simulink model "simulator_manual_MPC"  (R2025b)
settings: Solver=FixedStepAuto  StartTime=0.0  StopTime=100  FixedStep=0.01  RelTol=1e-3
values from neighbouring files (symbols this model uses):
  q0 = [0; 0; 0]    [model_init.m]    (also in test_model.m = x_test(1:3))
  qdot0 = [0;0;0]    [model_init.m]
  W_inv = inv(system_params.W)    [model_init.m]
undefined symbols (not defined in the file or in its folder): MPC_settings, P0, Q_kf, R_kf, system_params, x0
libraries: slpidlib x5
settings Model: Creator=Sigbjørn  LastModifiedBy=sig

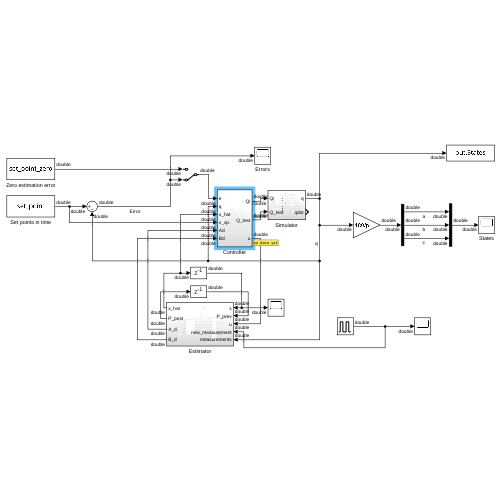
[thumbnail: Simulink's stored preview of the top-level diagram]
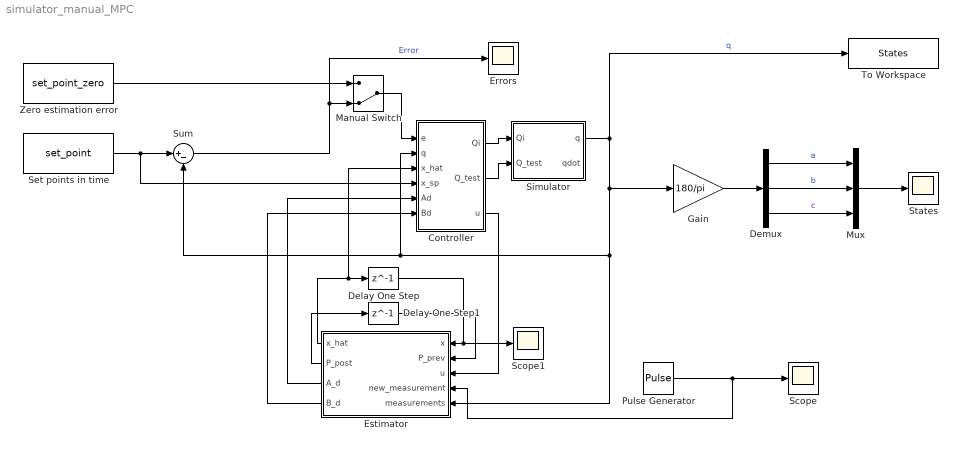
== system simulator_manual_MPC ==
  Controller : Subsystem
  Delay One Step : Delay  DelayLength=1  InitialCondition=x0
  Delay One Step1 : Delay  DelayLength=1  InitialCondition=P0
  Demux : Demux  Outputs=3
  Errors : Scope
      settings: ActiveDisplayYMinimum=-1.818734816898053E+64  ActiveDisplayYMaximum=2.7677532819561327E+63
  Estimator : Subsystem
      settings: PortSchema="{\"entries\":[{\"content\":{\"sides\":[{\"content\":{\"connectorIds\":[\"Out1\",\"Out2\",\"Out3\",\"Out4\"]},\"type\":\"ConnectorPlacement.EquallySpacedRectSide\",\"uuid\":\"f477ef40-4352-4d84-a45f-d7b8149414e1\"},{\"content\":{\"connectorIds\":[\"In1\",\"In2\",\"In3\",\"In4\",\"In5\"],\"side\":\"RIGHT\"},\"type\":\"ConnectorPlacement.EquallySpacedRectSide\",\"uuid\":\"8f29c47b-7819-47b7-a7db-3d460012710f\"},{\"content\":{\"side\":\"TOP\"},\"type\":\"ConnectorPlacement.EquallySpacedRectSide\",\"uuid\":\"6fcef62b-5cfa-49ba-93f4-5d540223ca0d\"}]},\"type\":\"ConnectorPlacement.EquallySpacedConnector\",\"uuid\":\"aa31ebfc-db05-4e23-be25-e9e271d34221\"}],\"packageUris\":[\"http://schema.mathworks.com/mf0/Connector/R2020b\"],\"version\":\"1.0\"}"
  Gain : Gain  Gain=180/pi
  Manual Switch : ManualSwitch  CurrentSetting=0
  Mux : Mux  Inputs=3
  Pulse Generator : DiscretePulseGenerator  PulseType=Time based  Period=0.1  PulseWidth=10
  Scope : Scope
      settings: ActiveDisplayYMinimum=-0.12499999999999997  ActiveDisplayYMaximum=1.125  DataLoggingVariableName=ScopeData11
  Scope1 : Scope
      settings: ActiveDisplayYMinimum=-0.00092258079795706066  ActiveDisplayYMaximum=0.0024721822800288758  DataLoggingVariableName=ScopeData13
  Set points in time : FromWorkspace  VariableName=set_point
  Simulator : Subsystem
  States : Scope
      settings: ActiveDisplayYMinimum=-1.5858058178956856E+65  ActiveDisplayYMaximum=1.0420582906175698E+66
  Sum : Sum  Inputs=|+-
  To Workspace : ToWorkspace  VariableName=States  SaveFormat=Timeseries  SampleTime=-1
  Zero estimation error : FromWorkspace  VariableName=set_point_zero
  wires:
  Controller/1(Qi) -> Simulator/1(Qi)
  Sum/1 -> Manual Switch/2, Errors/1  "Error"
  Simulator/1(q) -> Estimator/5(measurements), Controller/2(q), Sum/2, Gain/1, To Workspace/1  "q"
  Demux/1 -> Mux/1  "a"
  Demux/2 -> Mux/2  "b"
  Demux/3 -> Mux/3  "c"
  Zero estimation error/1 -> Manual Switch/1
  Manual Switch/1 -> Controller/1(e)
  Gain/1 -> Demux/1
  Mux/1 -> States/1
  Controller/2(Q_test) -> Simulator/2(Q_test)
  Controller/3(u) -> Estimator/3(u)
  Pulse Generator/1 -> Estimator/4(new_measurement), Scope/1
  Estimator/1(x_hat) -> Controller/3(x_hat), Delay One Step/1
  Estimator/2(P_post) -> Delay One Step1/1
  Delay One Step/1 -> Scope1/1, Estimator/1(x)
  Delay One Step1/1 -> Estimator/2(P_prev)
  Estimator/3(A_d) -> Controller/5(Ad)
  Estimator/4(B_d) -> Controller/6(Bd)
  Set points in time/1 -> Controller/4(x_sp), Sum/1

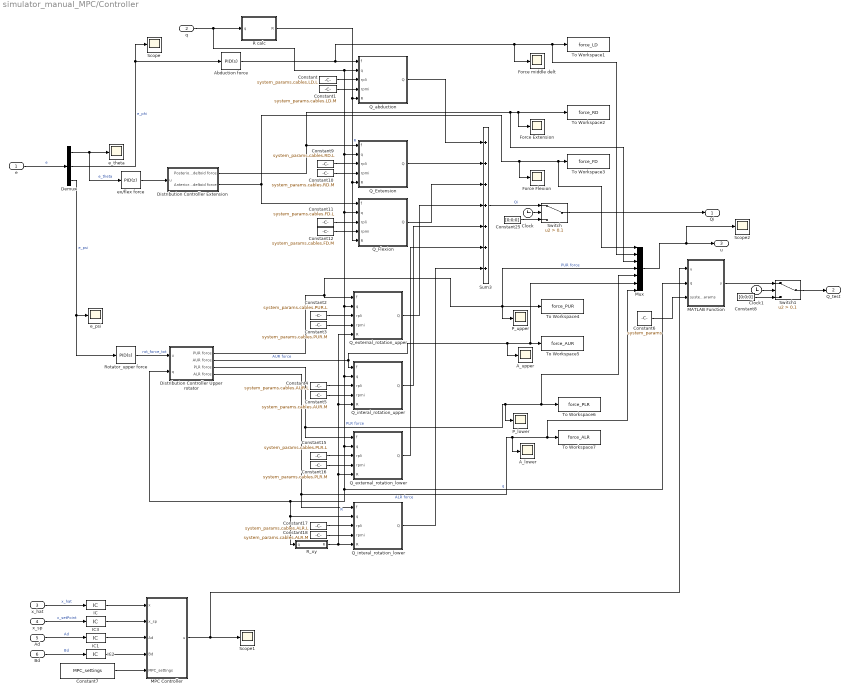
== system simulator_manual_MPC/Controller ==
  e : Inport
  q : Inport  Port=2
  x_hat : Inport  Port=3
  x_sp : Inport  Port=4
  Ad : Inport  Port=5
  Bd : Inport  Port=6
  A_lower : Scope
      settings: ActiveDisplayYMinimum=-66.70773  ActiveDisplayYMaximum=600.36959  DataLoggingVariableName=ScopeData3
  A_upper : Scope
      settings: ActiveDisplayYMinimum=-10.373094653487385  ActiveDisplayYMaximum=93.35785188138648  DataLoggingVariableName=ScopeData4
  Abduction force : slpidlib/PID Controller  Controller=PID  Form=Parallel  TimeDomain=Continuous-time  UseExternalTs=off  SampleTime=-1  IntegratorMethod=Forward Euler  FilterMethod=Forward Euler  ControllerParametersSource=internal  P=1  I=25  UseKiTs=off  D=5  UseExternalDerivativeSource=off  N=100  UseFilter=on  TunerSelectOption=Transfer Function Based (PID Tuner App)  InitialConditionSource=internal  InitialConditionForIntegrator=0  InitialConditionForFilter=0  DifferentiatorICPrevScaledInput=0  ExternalReset=none  TrackingMode=off  Kt=1  LimitOutput=on  SatLimitsSource=internal  UpperSaturationLimit=inf  LowerSaturationLimit=0  LinearizeAsGain=on  AntiWindupMode=none  Kb=1  LimitIntegrator=on  UpperIntegratorSaturationLimit=10000  LowerIntegratorSaturationLimit=0  POutMin=[]  POutMax=[]  IOutMin=[]  IOutMax=[]  DOutMin=[]  DOutMax=[]  NOutMin=[]  NOutMax=[]  SumOutMin=[]  SumOutMax=[]  SaturationOutMin=[]  SaturationOutMax=[]  PParamMin=[]  PParamMax=[]  IParamMin=[]  IParamMax=[]  DParamMin=[]  DParamMax=[]  NParamMin=[]  NParamMax=[]  KbParamMin=[]  KbParamMax=[]  KtParamMin=[]  KtParamMax=[]  KbOutMin=[]  KbOutMax=[]  KtOutMin=[]  KtOutMax=[]  IntegratorOutMin=[]  IntegratorOutMax=[]  FilterOutMin=[]  FilterOutMax=[]  SumI1OutMin=[]  SumI1OutMax=[]  SumI2OutMin=[]  SumI2OutMax=[]  SumI3OutMin=[]  SumI3OutMax=[]  SumI4OutMin=[]  SumI4OutMax=[]  SumDOutMin=[]  SumDOutMax=[]  DifferentiatorOutMin=[]  DifferentiatorOutMax=[]  FilterDiffOutCoefMin=[]  FilterDiffOutCoefMax=[]  ReciprocalOutMin=[]  ReciprocalOutMax=[]  SumDenOutMin=[]  SumDenOutMax=[]  SumNumOutMin=[]  SumNumOutMax=[]  DivideOutMin=[]  DivideOutMax=[]  UdiffTsProdOutMin=[]  UdiffTsProdOutMax=[]  NTsProdOutMin=[]  NTsProdOutMax=[]  UintegralTsProdOutMin=[]  UintegralTsProdOutMax=[]  UngainTsProdOutMin=[]  UngainTsProdOutMax=[]  ClampingZeroOutDataTypeStr=Inherit: Inherit via back propagation  ClampingZeroOutMin=[]  ClampingZeroOutMax=[]  FilterDenConstantOutDataTypeStr=Inherit: Inherit via back propagation  FilterDenConstantOutMin=[]  FilterDenConstantOutMax=[]  PCopyOutDataTypeStr=Inherit: Inherit via back propagation  PCopyOutMin=[]  PCopyOutMax=[]  NCopyOutDataTypeStr=Inherit: Inherit via back propagation  NCopyOutMin=[]  NCopyOutMax=[]  IntegratorContinuousStateAttributes=''  IntegratorStateMustResolveToSignalObject=off  IntegratorRTWStateStorageClass=Auto  FilterContinuousStateAttributes=''  FilterStateMustResolveToSignalObject=off  FilterRTWStateStorageClass=Auto  ParallelPVariant=InternalParameters  IdealPVariant=Disabled  IVariant=InternalParameters  DVariant=InternalParameters  IntegratorVariant=Continuous  SatVariant=Enabled  AWVariant=Passthrough  PCopyVariant=Disabled  TRVariant=Disabled  FdbkBlocksVariant=Forward  IdealPFdbkVariant=Disabled  SatFdbkVariant=Disabled  DerivativeFilterVariant=ContFilter  NVariant=InternalParameters  NCopyVariant=Disabled  FilterICVariant=InternalICsFilter  IntegratorICVariant=InternalICs  ExternalResetVariant=Disabled  TRSumVariant=Passthrough  SumFdbkVariant=Disabled  SumVariant=Sum_PID  TsampFilterVariant=InternalTs  TsampNgainVariant=Passthrough  TsampIntegralVariant=Disabled_SignalSpec  ExternalSaturationOutDataTypeStr=Inherit: Same as second input  DerivativeSourceVariant=ErrorSignal  PreIntVariant=InternalPreInt
  Clock : Clock
  Clock1 : Clock
  Constant : Constant  Value=system_params.cables.LD.L
  Constant1 : Constant  Value=system_params.cables.LD.M
  Constant10 : Constant  Value=system_params.cables.RD.M
  Constant11 : Constant  Value=system_params.cables.FD.L
  Constant12 : Constant  Value=system_params.cables.FD.M
  Constant15 : Constant  Value=system_params.cables.PLR.L
  Constant16 : Constant  Value=system_params.cables.PLR.M
  Constant17 : Constant  Value=system_params.cables.ALR.L
  Constant18 : Constant  Value=system_params.cables.ALR.M
  Constant2 : Constant  Value=system_params.cables.PUR.L
  Constant25 : Constant  Value=[0;0;0]
  Constant3 : Constant  Value=system_params.cables.PUR.M
  Constant4 : Constant  Value=system_params.cables.AUR.L
  Constant5 : Constant  Value=system_params.cables.AUR.M
  Constant6 : Constant  Value=system_params  OutDataTypeStr=Bus: System_params_bus
  Constant7 : Constant  Value=MPC_settings  OutDataTypeStr=Bus: MPCBus
  Constant8 : Constant  Value=[0;0;0]
  Constant9 : Constant  Value=system_params.cables.RD.L
  Demux : Demux  Outputs=3
  Distribution Controller Extension : Subsystem
  Distribution Controller Upper rotator : Subsystem
  Force Extension : Scope
      settings: ActiveDisplayYMinimum=-60.902718832950853  ActiveDisplayYMaximum=560.55994041701729
  Force Flexion : Scope
      settings: ActiveDisplayYMinimum=-3.2054062543658342  ActiveDisplayYMaximum=29.503154758790387  DataLoggingVariableName=ScopeData2
  Force middle delt : Scope
      settings: ActiveDisplayYMinimum=-835.43898  ActiveDisplayYMaximum=7657.08353  DataLoggingVariableName=ScopeData3
  IC : InitialCondition  Value=x0
  IC1 : InitialCondition  Value=zeros(6,6)
  IC2 : InitialCondition  Value=zeros(6,7)
  IC3 : InitialCondition  Value=zeros(3,1)
  MATLAB Function : MATLAB Function  TreatAsAtomicUnit=on
  MPC Controller : MATLAB Function  TreatAsAtomicUnit=on
  Mux : Mux  Inputs=7
  P_lower : Scope
      settings: ActiveDisplayYMinimum=-3.51093  ActiveDisplayYMaximum=31.5984  DataLoggingVariableName=ScopeData2
  P_upper : Scope
      settings: ActiveDisplayYMinimum=-0.42649  ActiveDisplayYMaximum=3.83839
  Q_Extension : MATLAB Function  TreatAsAtomicUnit=on
  Q_Flexion : MATLAB Function  TreatAsAtomicUnit=on
  Q_abduction : MATLAB Function  TreatAsAtomicUnit=on
  Q_external_rotation_lower : MATLAB Function  TreatAsAtomicUnit=on
  Q_external_rotation_upper : MATLAB Function  TreatAsAtomicUnit=on
  Q_interal_rotation_lower : MATLAB Function  TreatAsAtomicUnit=on
  Q_interal_rotation_upper : MATLAB Function  TreatAsAtomicUnit=on
  R calc : MATLAB Function  TreatAsAtomicUnit=on
  R_xy : MATLAB Function  TreatAsAtomicUnit=on
  Rotator_upper force : slpidlib/PID Controller  Controller=PID  Form=Parallel  TimeDomain=Continuous-time  UseExternalTs=off  SampleTime=-1  IntegratorMethod=Forward Euler  FilterMethod=Forward Euler  ControllerParametersSource=internal  P=100  I=200  UseKiTs=off  D=500  UseExternalDerivativeSource=off  N=100  UseFilter=on  TunerSelectOption=Transfer Function Based (PID Tuner App)  InitialConditionSource=internal  InitialConditionForIntegrator=0  InitialConditionForFilter=0  DifferentiatorICPrevScaledInput=0  ExternalReset=none  TrackingMode=off  Kt=1  LimitOutput=on  SatLimitsSource=internal  UpperSaturationLimit=inf  LowerSaturationLimit=-inf  LinearizeAsGain=on  AntiWindupMode=none  Kb=1  LimitIntegrator=on  UpperIntegratorSaturationLimit=inf  LowerIntegratorSaturationLimit=-inf  POutMin=[]  POutMax=[]  IOutMin=[]  IOutMax=[]  DOutMin=[]  DOutMax=[]  NOutMin=[]  NOutMax=[]  SumOutMin=[]  SumOutMax=[]  SaturationOutMin=[]  SaturationOutMax=[]  PParamMin=[]  PParamMax=[]  IParamMin=[]  IParamMax=[]  DParamMin=[]  DParamMax=[]  NParamMin=[]  NParamMax=[]  KbParamMin=[]  KbParamMax=[]  KtParamMin=[]  KtParamMax=[]  KbOutMin=[]  KbOutMax=[]  KtOutMin=[]  KtOutMax=[]  IntegratorOutMin=[]  IntegratorOutMax=[]  FilterOutMin=[]  FilterOutMax=[]  SumI1OutMin=[]  SumI1OutMax=[]  SumI2OutMin=[]  SumI2OutMax=[]  SumI3OutMin=[]  SumI3OutMax=[]  SumI4OutMin=[]  SumI4OutMax=[]  SumDOutMin=[]  SumDOutMax=[]  DifferentiatorOutMin=[]  DifferentiatorOutMax=[]  FilterDiffOutCoefMin=[]  FilterDiffOutCoefMax=[]  ReciprocalOutMin=[]  ReciprocalOutMax=[]  SumDenOutMin=[]  SumDenOutMax=[]  SumNumOutMin=[]  SumNumOutMax=[]  DivideOutMin=[]  DivideOutMax=[]  UdiffTsProdOutMin=[]  UdiffTsProdOutMax=[]  NTsProdOutMin=[]  NTsProdOutMax=[]  UintegralTsProdOutMin=[]  UintegralTsProdOutMax=[]  UngainTsProdOutMin=[]  UngainTsProdOutMax=[]  ClampingZeroOutDataTypeStr=Inherit: Inherit via back propagation  ClampingZeroOutMin=[]  ClampingZeroOutMax=[]  FilterDenConstantOutDataTypeStr=Inherit: Inherit via back propagation  FilterDenConstantOutMin=[]  FilterDenConstantOutMax=[]  PCopyOutDataTypeStr=Inherit: Inherit via back propagation  PCopyOutMin=[]  PCopyOutMax=[]  NCopyOutDataTypeStr=Inherit: Inherit via back propagation  NCopyOutMin=[]  NCopyOutMax=[]  IntegratorContinuousStateAttributes=''  IntegratorStateMustResolveToSignalObject=off  IntegratorRTWStateStorageClass=Auto  FilterContinuousStateAttributes=''  FilterStateMustResolveToSignalObject=off  FilterRTWStateStorageClass=Auto  ParallelPVariant=InternalParameters  IdealPVariant=Disabled  IVariant=InternalParameters  DVariant=InternalParameters  IntegratorVariant=Continuous  SatVariant=Enabled  AWVariant=Passthrough  PCopyVariant=Disabled  TRVariant=Disabled  FdbkBlocksVariant=Forward  IdealPFdbkVariant=Disabled  SatFdbkVariant=Disabled  DerivativeFilterVariant=ContFilter  NVariant=InternalParameters  NCopyVariant=Disabled  FilterICVariant=InternalICsFilter  IntegratorICVariant=InternalICs  ExternalResetVariant=Disabled  TRSumVariant=Passthrough  SumFdbkVariant=Disabled  SumVariant=Sum_PID  TsampFilterVariant=InternalTs  TsampNgainVariant=Passthrough  TsampIntegralVariant=Disabled_SignalSpec  ExternalSaturationOutDataTypeStr=Inherit: Same as second input  DerivativeSourceVariant=ErrorSignal  PreIntVariant=InternalPreInt
  Scope : Scope
      settings: ActiveDisplayYMinimum=-0.00043  ActiveDisplayYMaximum=5E-5  DataLoggingVariableName=ScopeData5
  Scope1 : Scope
      settings: ActiveDisplayYMinimum=-126637.74464504365  ActiveDisplayYMaximum=129137.74464504365  DataLoggingVariableName=ScopeData14
  Scope2 : Scope
      settings: ActiveDisplayYMinimum=-76.031922907283175  ActiveDisplayYMaximum=684.28730616554867  DataLoggingVariableName=ScopeData15
  Sum3 : Sum  Inputs=+++++++  InputSameDT=on  SaturateOnIntegerOverflow=on  OutDataTypeStr=Inherit: Same as first input
  Switch : Switch  Criteria=u2 > Threshold  Threshold=0.1  SaturateOnIntegerOverflow=off  InputSameDT=off
  Switch1 : Switch  Criteria=u2 > Threshold  Threshold=0.1  SaturateOnIntegerOverflow=off  InputSameDT=off
  To Workspace1 : ToWorkspace  VariableName=force_LD  SaveFormat=Timeseries  SampleTime=-1
  To Workspace2 : ToWorkspace  VariableName=force_RD  SaveFormat=Timeseries  SampleTime=-1
  To Workspace3 : ToWorkspace  VariableName=force_FD  SaveFormat=Timeseries  SampleTime=-1
  To Workspace4 : ToWorkspace  VariableName=force_PUR  SaveFormat=Timeseries  SampleTime=-1
  To Workspace5 : ToWorkspace  VariableName=force_AUR  SaveFormat=Timeseries  SampleTime=-1
  To Workspace6 : ToWorkspace  VariableName=force_PLR  SaveFormat=Timeseries  SampleTime=-1
  To Workspace7 : ToWorkspace  VariableName=force_ALR  SaveFormat=Timeseries  SampleTime=-1
  e_psi : Scope
      settings: ActiveDisplayYMinimum=-10.03144  ActiveDisplayYMaximum=67.48296  DataLoggingVariableName=ScopeData3
  e_theta : Scope
      settings: ActiveDisplayYMinimum=-0.00064  ActiveDisplayYMaximum=0.00057  DataLoggingVariableName=ScopeData6
  ex/flex force : slpidlib/PID Controller  Controller=PID  Form=Parallel  TimeDomain=Discrete-time  UseExternalTs=off  SampleTime=-1  IntegratorMethod=Forward Euler  FilterMethod=Forward Euler  ControllerParametersSource=internal  P=1  I=25  UseKiTs=off  D=5  UseExternalDerivativeSource=off  N=100  UseFilter=on  TunerSelectOption=Transfer Function Based (PID Tuner App)  InitialConditionSource=internal  InitialConditionForIntegrator=0  InitialConditionForFilter=0  DifferentiatorICPrevScaledInput=0  ExternalReset=none  TrackingMode=off  Kt=1  LimitOutput=on  SatLimitsSource=internal  UpperSaturationLimit=inf  LowerSaturationLimit=-inf  LinearizeAsGain=on  AntiWindupMode=none  Kb=1  LimitIntegrator=on  UpperIntegratorSaturationLimit=inf  LowerIntegratorSaturationLimit=-inf  POutMin=[]  POutMax=[]  IOutMin=[]  IOutMax=[]  DOutMin=[]  DOutMax=[]  NOutMin=[]  NOutMax=[]  SumOutMin=[]  SumOutMax=[]  SaturationOutMin=[]  SaturationOutMax=[]  PParamMin=[]  PParamMax=[]  IParamMin=[]  IParamMax=[]  DParamMin=[]  DParamMax=[]  NParamMin=[]  NParamMax=[]  KbParamMin=[]  KbParamMax=[]  KtParamMin=[]  KtParamMax=[]  KbOutMin=[]  KbOutMax=[]  KtOutMin=[]  KtOutMax=[]  IntegratorOutMin=[]  IntegratorOutMax=[]  FilterOutMin=[]  FilterOutMax=[]  SumI1OutMin=[]  SumI1OutMax=[]  SumI2OutMin=[]  SumI2OutMax=[]  SumI3OutMin=[]  SumI3OutMax=[]  SumI4OutMin=[]  SumI4OutMax=[]  SumDOutMin=[]  SumDOutMax=[]  DifferentiatorOutMin=[]  DifferentiatorOutMax=[]  FilterDiffOutCoefMin=[]  FilterDiffOutCoefMax=[]  ReciprocalOutMin=[]  ReciprocalOutMax=[]  SumDenOutMin=[]  SumDenOutMax=[]  SumNumOutMin=[]  SumNumOutMax=[]  DivideOutMin=[]  DivideOutMax=[]  UdiffTsProdOutMin=[]  UdiffTsProdOutMax=[]  NTsProdOutMin=[]  NTsProdOutMax=[]  UintegralTsProdOutMin=[]  UintegralTsProdOutMax=[]  UngainTsProdOutMin=[]  UngainTsProdOutMax=[]  ClampingZeroOutDataTypeStr=Inherit: Inherit via back propagation  ClampingZeroOutMin=[]  ClampingZeroOutMax=[]  FilterDenConstantOutDataTypeStr=Inherit: Inherit via back propagation  FilterDenConstantOutMin=[]  FilterDenConstantOutMax=[]  PCopyOutDataTypeStr=Inherit: Inherit via back propagation  PCopyOutMin=[]  PCopyOutMax=[]  NCopyOutDataTypeStr=Inherit: Inherit via back propagation  NCopyOutMin=[]  NCopyOutMax=[]  IntegratorContinuousStateAttributes=''  IntegratorStateMustResolveToSignalObject=off  IntegratorRTWStateStorageClass=Auto  FilterContinuousStateAttributes=''  FilterStateMustResolveToSignalObject=off  FilterRTWStateStorageClass=Auto  ParallelPVariant=InternalParameters  IdealPVariant=Disabled  IVariant=InternalParameters  DVariant=InternalParameters  IntegratorVariant=Discrete  SatVariant=Enabled  AWVariant=Passthrough  PCopyVariant=Disabled  TRVariant=Disabled  FdbkBlocksVariant=Forward  IdealPFdbkVariant=Disabled  SatFdbkVariant=Disabled  DerivativeFilterVariant=ForwardEulerFilter  NVariant=InternalParameters  NCopyVariant=Disabled  FilterICVariant=InternalICsFilter  IntegratorICVariant=InternalICs  ExternalResetVariant=Disabled  TRSumVariant=Passthrough  SumFdbkVariant=Disabled  SumVariant=Sum_PID  TsampFilterVariant=InternalTs  TsampNgainVariant=Passthrough  TsampIntegralVariant=Disabled_SignalSpec  ExternalSaturationOutDataTypeStr=Inherit: Same as second input  DerivativeSourceVariant=ErrorSignal  PreIntVariant=InternalPreInt
  Qi : Outport
  Q_test : Outport  Port=2
  u : Outport  Port=3
  wires:
  q/1 -> Q_abduction/2(q), Q_Extension/2(q), Q_Flexion/2(q), MATLAB Function/2(q), Q_interal_rotation_lower/2(q), R_xy/1(q), Distribution Controller Upper rotator/2(q), Q_external_rotation_lower/2(q), Q_interal_rotation_upper/2(q), Q_external_rotation_upper/2(q), R calc/1(q)  "q"
  R calc/1(R) -> Q_Extension/5(R), Q_Flexion/5(R), Q_abduction/5(R)  "R"
  Constant/1 -> Q_abduction/3(rpli)
  Constant1/1 -> Q_abduction/4(rpmi)
  Sum3/1 -> Switch/1  "Qi"
  Demux/1 -> ex/flex force/1, e_theta/1  "e_theta"
  Demux/2 -> Scope/1, Abduction force/1  "e_phi"
  Demux/3 -> Rotator_upper force/1, e_psi/1  "e_psi"
  Constant2/1 -> Q_external_rotation_upper/3(rpli)
  Constant3/1 -> Q_external_rotation_upper/4(rpmi)
  Constant4/1 -> Q_interal_rotation_upper/3(rpli)
  Constant5/1 -> Q_interal_rotation_upper/4(rpmi)
  Q_abduction/1(Q) -> Sum3/1
  Q_interal_rotation_upper/1(Q) -> Sum3/5
  Q_external_rotation_upper/1(Q) -> Sum3/4
  Rotator_upper force/1 -> Distribution Controller Upper rotator/1(u)  "rot_force_tot"
  ex/flex force/1 -> Distribution Controller Extension/1(u)
  Constant9/1 -> Q_Extension/3(rpli)
  Constant10/1 -> Q_Extension/4(rpmi)
  Constant11/1 -> Q_Flexion/3(rpli)
  Constant12/1 -> Q_Flexion/4(rpmi)
  Q_Flexion/1(Q) -> Sum3/3
  Q_Extension/1(Q) -> Sum3/2
  Abduction force/1 -> Force middle delt/1, Mux/2, To Workspace1/1, Q_abduction/1(f)
  Distribution Controller Extension/1(Posterior deltoid force) -> Mux/3, To Workspace2/1, Force Extension/1, Q_Extension/1(f)
  Distribution Controller Extension/2(Anterior deltoid force) -> Q_Flexion/1(f), Mux/1, To Workspace3/1, Force Flexion/1
  Q_external_rotation_lower/1(Q) -> Sum3/6
  Q_interal_rotation_lower/1(Q) -> Sum3/7
  Constant15/1 -> Q_external_rotation_lower/3(rpli)
  Constant16/1 -> Q_external_rotation_lower/4(rpmi)
  Constant17/1 -> Q_interal_rotation_lower/3(rpli)
  Constant18/1 -> Q_interal_rotation_lower/4(rpmi)
  e/1 -> Demux/1  "e"
  Clock/1 -> Switch/2
  Constant25/1 -> Switch/3
  Switch/1 -> Qi/1
  Distribution Controller Upper rotator/4(ALR force) -> Mux/7, To Workspace7/1, A_lower/1, Q_interal_rotation_lower/1(f)  "ALR force"
  Distribution Controller Upper rotator/3(PLR force) -> Mux/5, To Workspace6/1, P_lower/1, Q_external_rotation_lower/1(f)  "PLR force"
  Distribution Controller Upper rotator/2(AUR force) -> A_upper/1, Mux/6, To Workspace5/1, Q_interal_rotation_upper/1(f)  "AUR force"
  Distribution Controller Upper rotator/1(PUR force) -> Mux/4, To Workspace4/1, P_upper/1, Q_external_rotation_upper/1(f)  "PUR force"
  R_xy/1(R) -> Q_external_rotation_upper/5(R), Q_interal_rotation_upper/5(R), Q_external_rotation_lower/5(R), Q_interal_rotation_lower/5(R)  "R"
  Mux/1 -> Scope2/1, u/1
  MATLAB Function/1(y) -> Switch1/1
  Constant6/1 -> MATLAB Function/3(system_params)
  x_hat/1 -> IC/1  "x_hat"
  Ad/1 -> IC1/1  "Ad"
  Bd/1 -> IC2/1  "Bd"
  Constant7/1 -> MPC Controller/5(MPC_settings)
  MPC Controller/1(u) -> MATLAB Function/1(u), Scope1/1
  x_sp/1 -> IC3/1  "x_setPoint"
  Constant8/1 -> Switch1/3
  Switch1/1 -> Q_test/1
  Clock1/1 -> Switch1/2
  IC/1 -> MPC Controller/1(x)
  IC1/1 -> MPC Controller/3(Ad)
  IC2/1 -> MPC Controller/4(Bd)
  IC3/1 -> MPC Controller/2(x_sp)

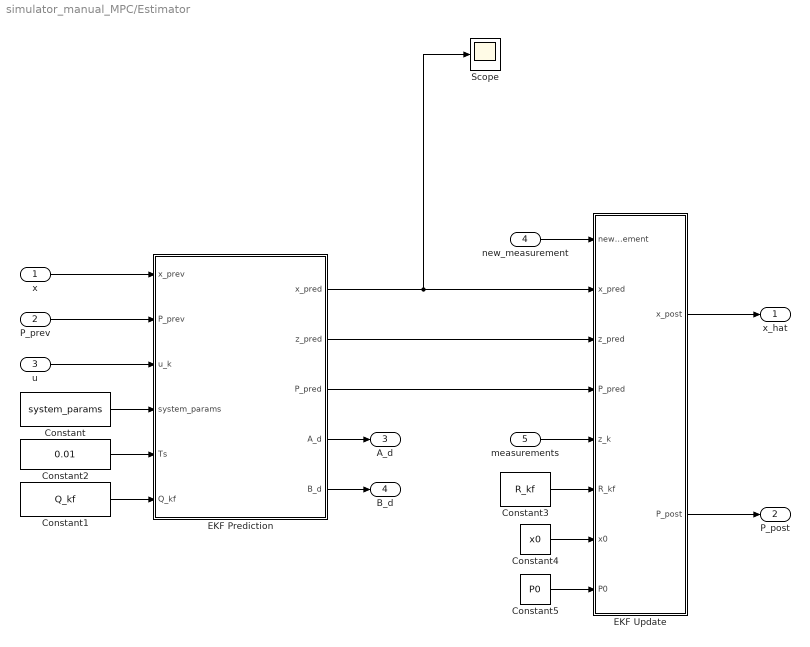
== system simulator_manual_MPC/Estimator ==
  x : Inport
  P_prev : Inport  Port=2
  u : Inport  Port=3
  new_measurement : Inport  Port=4
  measurements : Inport  Port=5
  Constant : Constant  Value=system_params  OutDataTypeStr=Bus: System_params_bus
  Constant1 : Constant  Value=Q_kf
  Constant2 : Constant  Value=0.01
  Constant3 : Constant  Value=R_kf
  Constant4 : Constant  Value=x0
  Constant5 : Constant  Value=P0
  EKF Prediction : MATLAB Function  TreatAsAtomicUnit=on
  EKF Update : MATLAB Function  TreatAsAtomicUnit=on
  Scope : Scope
      settings: ActiveDisplayYMinimum=-0.013878209930986719  ActiveDisplayYMaximum=0.011656451557926608  DataLoggingVariableName=ScopeData12
  x_hat : Outport
  P_post : Outport  Port=2
  A_d : Outport  Port=3
  B_d : Outport  Port=4
  wires:
  x/1 -> EKF Prediction/1(x_prev)
  EKF Update/1(x_post) -> x_hat/1
  u/1 -> EKF Prediction/3(u_k)
  P_prev/1 -> EKF Prediction/2(P_prev)
  Constant/1 -> EKF Prediction/4(system_params)
  Constant1/1 -> EKF Prediction/6(Q_kf)
  Constant2/1 -> EKF Prediction/5(Ts)
  EKF Prediction/1(x_pred) -> Scope/1, EKF Update/2(x_pred)
  EKF Prediction/2(z_pred) -> EKF Update/3(z_pred)
  EKF Prediction/3(P_pred) -> EKF Update/4(P_pred)
  EKF Prediction/4(A_d) -> A_d/1
  EKF Prediction/5(B_d) -> B_d/1
  new_measurement/1 -> EKF Update/1(new_measurement)
  EKF Update/2(P_post) -> P_post/1
  Constant3/1 -> EKF Update/6(R_kf)
  measurements/1 -> EKF Update/5(z_k)
  Constant4/1 -> EKF Update/7(x0)
  Constant5/1 -> EKF Update/8(P0)

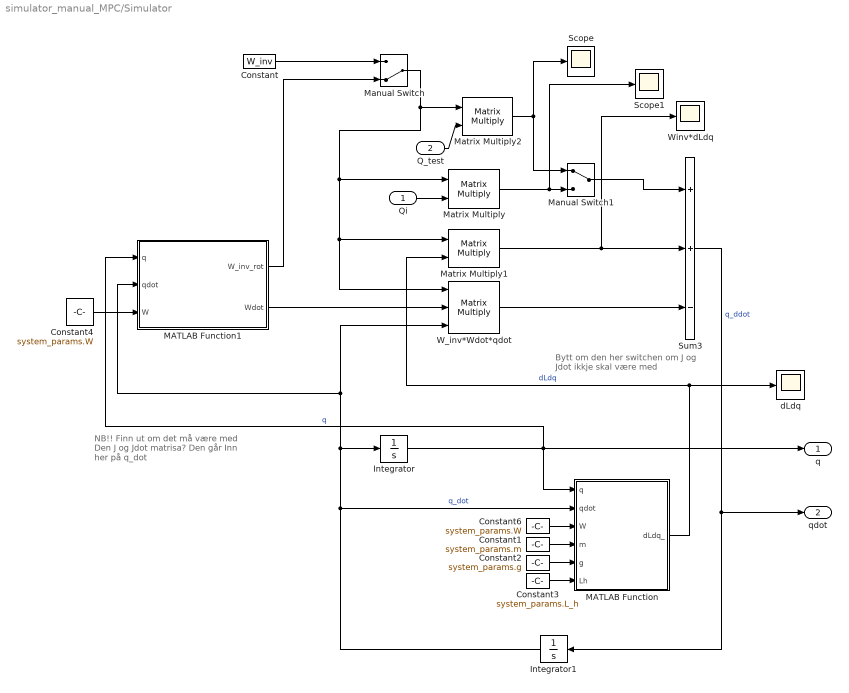
== system simulator_manual_MPC/Simulator ==
  note: Bytt om den her switchen
      | om J og Jdot ikkje skal være med
  note: NB!! Finn ut om det må være med
      | Den J og Jdot matrisa? Den går
      | Inn her på q_dot
  Qi : Inport
  Q_test : Inport  Port=2
  Constant : Constant  Value=W_inv
  Constant1 : Constant  Value=system_params.m
  Constant2 : Constant  Value=system_params.g
  Constant3 : Constant  Value=system_params.L_h
  Constant4 : Constant  Value=system_params.W
  Constant6 : Constant  Value=system_params.W
  Integrator : Integrator  InitialCondition=q0
  Integrator1 : Integrator  InitialCondition=qdot0
  MATLAB Function : MATLAB Function  TreatAsAtomicUnit=on
  MATLAB Function1 : MATLAB Function  TreatAsAtomicUnit=on
  Manual Switch : ManualSwitch  CurrentSetting=0
  Manual Switch1 : ManualSwitch
  Matrix Multiply : Product  Multiplication=Matrix(*)
  Matrix Multiply1 : Product  Multiplication=Matrix(*)
  Matrix Multiply2 : Product  Multiplication=Matrix(*)
  Scope : Scope
      settings: ActiveDisplayYMinimum=-7.018265804855659  ActiveDisplayYMaximum=14.492290543082335  DataLoggingVariableName=ScopeData9
  Scope1 : Scope
      settings: ActiveDisplayYMinimum=-3.4678856908682762  ActiveDisplayYMaximum=14.936630459412994  DataLoggingVariableName=ScopeData10
  Sum3 : Sum  Inputs=++-  InputSameDT=on  SaturateOnIntegerOverflow=on  OutDataTypeStr=Inherit: Same as first input
  W_inv*Wdot*qdot : Product  Inputs=3  Multiplication=Matrix(*)
  Winv*dLdq : Scope
      settings: ActiveDisplayYMinimum=-16798.22736  ActiveDisplayYMaximum=5519.64257
  dLdq : Scope
      settings: ActiveDisplayYMinimum=-257.99457  ActiveDisplayYMaximum=243.23473  DataLoggingVariableName=ScopeData2
  q : Outport
  qdot : Outport  Port=2
  wires:
  Qi/1 -> Matrix Multiply/2
  Constant1/1 -> MATLAB Function/4(m)
  Constant2/1 -> MATLAB Function/5(g)
  Constant3/1 -> MATLAB Function/6(Lh)
  Integrator/1 -> MATLAB Function1/1(q), q/1, MATLAB Function/1(q)  "q"
  Integrator1/1 -> W_inv*Wdot*qdot/3, MATLAB Function1/2(qdot), Integrator/1, MATLAB Function/2(qdot)  "q_dot"
  MATLAB Function/1(dLdq_) -> dLdq/1, Matrix Multiply1/2  "dLdq"
  Sum3/1 -> qdot/1, Integrator1/1  "q_ddot"
  Matrix Multiply/1 -> Manual Switch1/2, Scope1/1
  Matrix Multiply1/1 -> Winv*dLdq/1, Sum3/2
  Constant/1 -> Manual Switch/1
  MATLAB Function1/2(Wdot) -> W_inv*Wdot*qdot/2
  MATLAB Function1/1(W_inv_rot) -> Manual Switch/2
  Manual Switch/1 -> Matrix Multiply2/1, W_inv*Wdot*qdot/1, Matrix Multiply1/1, Matrix Multiply/1
  Constant4/1 -> MATLAB Function1/3(W)
  W_inv*Wdot*qdot/1 -> Sum3/3
  Constant6/1 -> MATLAB Function/3(W)
  Matrix Multiply2/1 -> Manual Switch1/1, Scope/1
  Q_test/1 -> Matrix Multiply2/2
  Manual Switch1/1 -> Sum3/1

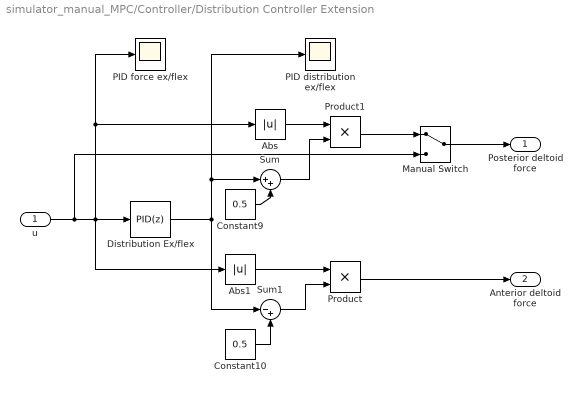
== system simulator_manual_MPC/Controller/Distribution Controller Extension ==
  u : Inport
  Abs : Abs  SaturateOnIntegerOverflow=off
  Abs1 : Abs  SaturateOnIntegerOverflow=off
  Constant10 : Constant  Value=0.5
  Constant9 : Constant  Value=0.5
  Distribution Ex/flex : slpidlib/PID Controller  Controller=PID  Form=Parallel  TimeDomain=Discrete-time  UseExternalTs=off  SampleTime=-1  IntegratorMethod=Forward Euler  FilterMethod=Forward Euler  ControllerParametersSource=internal  P=100  I=0  UseKiTs=off  D=0  UseExternalDerivativeSource=off  N=100  UseFilter=on  TunerSelectOption=Transfer Function Based (PID Tuner App)  InitialConditionSource=internal  InitialConditionForIntegrator=0  InitialConditionForFilter=0  DifferentiatorICPrevScaledInput=0  ExternalReset=none  TrackingMode=off  Kt=1  LimitOutput=on  SatLimitsSource=internal  UpperSaturationLimit=0.45  LowerSaturationLimit=-0.45  LinearizeAsGain=on  AntiWindupMode=none  Kb=1  LimitIntegrator=on  UpperIntegratorSaturationLimit=10  LowerIntegratorSaturationLimit=0  POutMin=[]  POutMax=[]  IOutMin=[]  IOutMax=[]  DOutMin=[]  DOutMax=[]  NOutMin=[]  NOutMax=[]  SumOutMin=[]  SumOutMax=[]  SaturationOutMin=[]  SaturationOutMax=[]  PParamMin=[]  PParamMax=[]  IParamMin=[]  IParamMax=[]  DParamMin=[]  DParamMax=[]  NParamMin=[]  NParamMax=[]  KbParamMin=[]  KbParamMax=[]  KtParamMin=[]  KtParamMax=[]  KbOutMin=[]  KbOutMax=[]  KtOutMin=[]  KtOutMax=[]  IntegratorOutMin=[]  IntegratorOutMax=[]  FilterOutMin=[]  FilterOutMax=[]  SumI1OutMin=[]  SumI1OutMax=[]  SumI2OutMin=[]  SumI2OutMax=[]  SumI3OutMin=[]  SumI3OutMax=[]  SumI4OutMin=[]  SumI4OutMax=[]  SumDOutMin=[]  SumDOutMax=[]  DifferentiatorOutMin=[]  DifferentiatorOutMax=[]  FilterDiffOutCoefMin=[]  FilterDiffOutCoefMax=[]  ReciprocalOutMin=[]  ReciprocalOutMax=[]  SumDenOutMin=[]  SumDenOutMax=[]  SumNumOutMin=[]  SumNumOutMax=[]  DivideOutMin=[]  DivideOutMax=[]  UdiffTsProdOutMin=[]  UdiffTsProdOutMax=[]  NTsProdOutMin=[]  NTsProdOutMax=[]  UintegralTsProdOutMin=[]  UintegralTsProdOutMax=[]  UngainTsProdOutMin=[]  UngainTsProdOutMax=[]  ClampingZeroOutDataTypeStr=Inherit: Inherit via back propagation  ClampingZeroOutMin=[]  ClampingZeroOutMax=[]  FilterDenConstantOutDataTypeStr=Inherit: Inherit via back propagation  FilterDenConstantOutMin=[]  FilterDenConstantOutMax=[]  PCopyOutDataTypeStr=Inherit: Inherit via back propagation  PCopyOutMin=[]  PCopyOutMax=[]  NCopyOutDataTypeStr=Inherit: Inherit via back propagation  NCopyOutMin=[]  NCopyOutMax=[]  IntegratorContinuousStateAttributes=''  IntegratorStateMustResolveToSignalObject=off  IntegratorRTWStateStorageClass=Auto  FilterContinuousStateAttributes=''  FilterStateMustResolveToSignalObject=off  FilterRTWStateStorageClass=Auto  ParallelPVariant=InternalParameters  IdealPVariant=Disabled  IVariant=InternalParameters  DVariant=InternalParameters  IntegratorVariant=Discrete  SatVariant=Enabled  AWVariant=Passthrough  PCopyVariant=Disabled  TRVariant=Disabled  FdbkBlocksVariant=Forward  IdealPFdbkVariant=Disabled  SatFdbkVariant=Disabled  DerivativeFilterVariant=ForwardEulerFilter  NVariant=InternalParameters  NCopyVariant=Disabled  FilterICVariant=InternalICsFilter  IntegratorICVariant=InternalICs  ExternalResetVariant=Disabled  TRSumVariant=Passthrough  SumFdbkVariant=Disabled  SumVariant=Sum_PID  TsampFilterVariant=InternalTs  TsampNgainVariant=Passthrough  TsampIntegralVariant=Disabled_SignalSpec  ExternalSaturationOutDataTypeStr=Inherit: Same as second input  DerivativeSourceVariant=ErrorSignal  PreIntVariant=InternalPreInt
  Manual Switch : ManualSwitch
  PID distribution ex/flex : Scope
      settings: ActiveDisplayYMinimum=-0.5625  ActiveDisplayYMaximum=0.5625  DataLoggingVariableName=ScopeData8
  PID force ex/flex : Scope
      settings: ActiveDisplayYMinimum=-0.16319  ActiveDisplayYMaximum=0.10006  DataLoggingVariableName=ScopeData7
  Product : Product
  Product1 : Product
  Sum : Sum  Inputs=|++
  Sum1 : Sum  Inputs=|-+
  Posterior deltoid force : Outport
  Anterior deltoid force : Outport  Port=2
  wires:
  Constant10/1 -> Sum1/2
  u/1 -> Manual Switch/2, Distribution Ex/flex/1, PID force ex/flex/1, Abs/1, Abs1/1
  Distribution Ex/flex/1 -> Sum1/1, PID distribution ex/flex/1, Sum/1
  Abs1/1 -> Product/1
  Sum/1 -> Product1/2
  Sum1/1 -> Product/2
  Abs/1 -> Product1/1
  Constant9/1 -> Sum/2
  Product1/1 -> Manual Switch/1
  Product/1 -> Anterior deltoid force/1
  Manual Switch/1 -> Posterior deltoid force/1

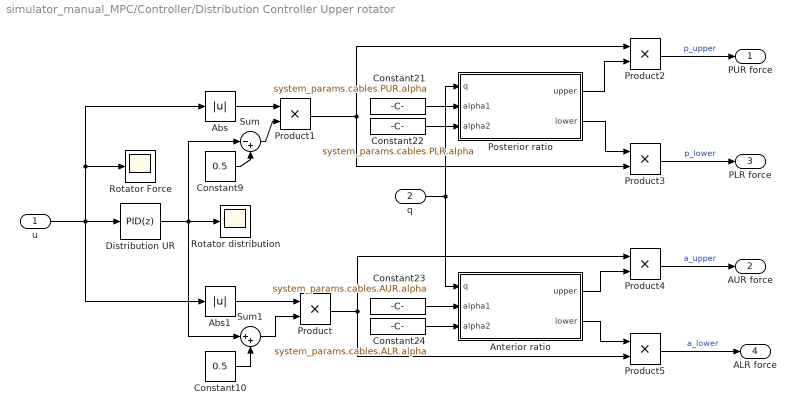
== system simulator_manual_MPC/Controller/Distribution Controller Upper rotator ==
  u : Inport
  q : Inport  Port=2
  Abs : Abs  SaturateOnIntegerOverflow=off
  Abs1 : Abs  SaturateOnIntegerOverflow=off
  Anterior ratio : MATLAB Function  TreatAsAtomicUnit=on
  Constant10 : Constant  Value=0.5
  Constant21 : Constant  Value=system_params.cables.PUR.alpha
  Constant22 : Constant  Value=system_params.cables.PLR.alpha
  Constant23 : Constant  Value=system_params.cables.AUR.alpha
  Constant24 : Constant  Value=system_params.cables.ALR.alpha
  Constant9 : Constant  Value=0.5
  Distribution UR : slpidlib/PID Controller  Controller=PID  Form=Parallel  TimeDomain=Discrete-time  UseExternalTs=off  SampleTime=-1  IntegratorMethod=Forward Euler  FilterMethod=Forward Euler  ControllerParametersSource=internal  P=100  I=0  UseKiTs=off  D=0  UseExternalDerivativeSource=off  N=100  UseFilter=on  TunerSelectOption=Transfer Function Based (PID Tuner App)  InitialConditionSource=internal  InitialConditionForIntegrator=0  InitialConditionForFilter=0  DifferentiatorICPrevScaledInput=0  ExternalReset=none  TrackingMode=off  Kt=1  LimitOutput=on  SatLimitsSource=internal  UpperSaturationLimit=0.45  LowerSaturationLimit=-0.45  LinearizeAsGain=on  AntiWindupMode=none  Kb=1  LimitIntegrator=on  UpperIntegratorSaturationLimit=10  LowerIntegratorSaturationLimit=0  POutMin=[]  POutMax=[]  IOutMin=[]  IOutMax=[]  DOutMin=[]  DOutMax=[]  NOutMin=[]  NOutMax=[]  SumOutMin=[]  SumOutMax=[]  SaturationOutMin=[]  SaturationOutMax=[]  PParamMin=[]  PParamMax=[]  IParamMin=[]  IParamMax=[]  DParamMin=[]  DParamMax=[]  NParamMin=[]  NParamMax=[]  KbParamMin=[]  KbParamMax=[]  KtParamMin=[]  KtParamMax=[]  KbOutMin=[]  KbOutMax=[]  KtOutMin=[]  KtOutMax=[]  IntegratorOutMin=[]  IntegratorOutMax=[]  FilterOutMin=[]  FilterOutMax=[]  SumI1OutMin=[]  SumI1OutMax=[]  SumI2OutMin=[]  SumI2OutMax=[]  SumI3OutMin=[]  SumI3OutMax=[]  SumI4OutMin=[]  SumI4OutMax=[]  SumDOutMin=[]  SumDOutMax=[]  DifferentiatorOutMin=[]  DifferentiatorOutMax=[]  FilterDiffOutCoefMin=[]  FilterDiffOutCoefMax=[]  ReciprocalOutMin=[]  ReciprocalOutMax=[]  SumDenOutMin=[]  SumDenOutMax=[]  SumNumOutMin=[]  SumNumOutMax=[]  DivideOutMin=[]  DivideOutMax=[]  UdiffTsProdOutMin=[]  UdiffTsProdOutMax=[]  NTsProdOutMin=[]  NTsProdOutMax=[]  UintegralTsProdOutMin=[]  UintegralTsProdOutMax=[]  UngainTsProdOutMin=[]  UngainTsProdOutMax=[]  ClampingZeroOutDataTypeStr=Inherit: Inherit via back propagation  ClampingZeroOutMin=[]  ClampingZeroOutMax=[]  FilterDenConstantOutDataTypeStr=Inherit: Inherit via back propagation  FilterDenConstantOutMin=[]  FilterDenConstantOutMax=[]  PCopyOutDataTypeStr=Inherit: Inherit via back propagation  PCopyOutMin=[]  PCopyOutMax=[]  NCopyOutDataTypeStr=Inherit: Inherit via back propagation  NCopyOutMin=[]  NCopyOutMax=[]  IntegratorContinuousStateAttributes=''  IntegratorStateMustResolveToSignalObject=off  IntegratorRTWStateStorageClass=Auto  FilterContinuousStateAttributes=''  FilterStateMustResolveToSignalObject=off  FilterRTWStateStorageClass=Auto  ParallelPVariant=InternalParameters  IdealPVariant=Disabled  IVariant=InternalParameters  DVariant=InternalParameters  IntegratorVariant=Discrete  SatVariant=Enabled  AWVariant=Passthrough  PCopyVariant=Disabled  TRVariant=Disabled  FdbkBlocksVariant=Forward  IdealPFdbkVariant=Disabled  SatFdbkVariant=Disabled  DerivativeFilterVariant=ForwardEulerFilter  NVariant=InternalParameters  NCopyVariant=Disabled  FilterICVariant=InternalICsFilter  IntegratorICVariant=InternalICs  ExternalResetVariant=Disabled  TRSumVariant=Passthrough  SumFdbkVariant=Disabled  SumVariant=Sum_PID  TsampFilterVariant=InternalTs  TsampNgainVariant=Passthrough  TsampIntegralVariant=Disabled_SignalSpec  ExternalSaturationOutDataTypeStr=Inherit: Same as second input  DerivativeSourceVariant=ErrorSignal  PreIntVariant=InternalPreInt
  Posterior ratio : MATLAB Function  TreatAsAtomicUnit=on
  Product{,1..5} (6 alike) : Product
  Rotator Force : Scope
      settings: ActiveDisplayYMinimum=-13.1342  ActiveDisplayYMaximum=118.2078  DataLoggingVariableName=ScopeData5
  Rotator distribution : Scope
  Sum : Sum  Inputs=|-+
  Sum1 : Sum  Inputs=|++
  PUR force : Outport
  AUR force : Outport  Port=2
  PLR force : Outport  Port=3
  ALR force : Outport  Port=4
  wires:
  Constant10/1 -> Sum1/2
  u/1 -> Abs1/1, Distribution UR/1, Rotator Force/1, Abs/1
  Distribution UR/1 -> Rotator distribution/1, Sum1/1, Sum/1
  Abs1/1 -> Product/1
  Sum/1 -> Product1/2
  Sum1/1 -> Product/2
  Abs/1 -> Product1/1
  Constant9/1 -> Sum/2
  Posterior ratio/1(upper) -> Product2/2
  Constant24/1 -> Anterior ratio/3(alpha2)
  Constant23/1 -> Anterior ratio/2(alpha1)
  Anterior ratio/2(lower) -> Product5/1
  Product5/1 -> ALR force/1  "a_lower"
  q/1 -> Posterior ratio/1(q), Anterior ratio/1(q)
  Constant21/1 -> Posterior ratio/2(alpha1)
  Constant22/1 -> Posterior ratio/3(alpha2)
  Anterior ratio/1(upper) -> Product4/2
  Product/1 -> Product4/1, Product5/2
  Product2/1 -> PUR force/1  "p_upper"
  Posterior ratio/2(lower) -> Product3/1
  Product4/1 -> AUR force/1  "a_upper"
  Product1/1 -> Product3/2, Product2/1
  Product3/1 -> PLR force/1  "p_lower"

== matlab function simulator_manual_MPC/Controller/R_xy ==
  data: q input; R output
function R = fcn(q)
R = Rot_xy(q);

== matlab function simulator_manual_MPC/Controller/Q_external_rotation_lower ==
  data: f input; Q output; q input; rpli input; rpmi input; R input
function Q = fcn(f, q, rpli, rpmi, R)

Q = Qi(f, q, rpli, rpmi, R);

== matlab function simulator_manual_MPC/Controller/Q_interal_rotation_lower ==
  data: f input; Q output; q input; rpli input; rpmi input; R input
function Q = fcn(f, q, rpli, rpmi, R)

Q = Qi(f, q, rpli, rpmi, R);

== matlab function simulator_manual_MPC/Controller/MATLAB Function ==
  settings: updateMethod=DISCRETE  sampleTime=dt
  data: u input; y output; q input; system_params input
function y = fcn(u,q,system_params)
y = Q_force_calc(u, q, system_params);

== matlab function simulator_manual_MPC/Estimator/EKF Prediction ==
  data: x_prev input size=[6 1]; x_pred output; P_prev input size=[6 6]; u_k input; z_pred output; P_pred output; A_d output; B_d output; system_params input; Ts input; Q_kf input
function [x_pred, z_pred, P_pred, A_d, B_d] = fcn(x_prev, P_prev, u_k, system_params, Ts, Q_kf)

[x_pred, z_pred, P_pred, A_d, B_d] = EKF_pred(x_prev, P_prev, u_k, system_params, Ts, Q_kf);

== matlab function simulator_manual_MPC/Controller/Distribution Controller Upper rotator/Anterior ratio ==
  data: q input; upper output; alpha1 input; alpha2 input; lower output
function [upper, lower] = ul_rat(q, alpha1, alpha2)

[upper, lower] = ul_ratio(q, alpha1, alpha2);

== matlab function simulator_manual_MPC/Simulator/MATLAB Function1 ==
  data: q input; qdot input; W input; W_inv_rot output; Wdot output
function [W_inv_rot, Wdot] = W_Wdot_call(q, qdot, W)

[W_inv_rot, Wdot] = W_Wdot(q, qdot, W);

== matlab function simulator_manual_MPC/Controller/Distribution Controller Upper rotator/Posterior ratio ==
  data: q input; upper output; alpha1 input; alpha2 input; lower output
function [upper, lower] = ul_rat(q, alpha1, alpha2)

[upper, lower] = ul_ratio(q, alpha1, alpha2);

== matlab function simulator_manual_MPC/Estimator/EKF Update ==
  data: new_measurement input; x_pred input size=[6 1]; z_pred input; x_post output size=[6,1]; P_pred input double size=[6 6]; z_k input; R_kf input; P_post output; x0 input; P0 input
function [x_post,P_post] = fcn(new_measurement, x_pred, z_pred, P_pred, z_k, R_kf, x0, P0)

persistent isInitialized
if isempty(isInitialized)
    x_pred = x0;
    P_pred = P0;
    isInitialized = true;
end

if new_measurement
    [x_post,P_post] = EKF_upd(x_pred, P_pred, z_pred, z_k, R_kf);
else
    x_post = x_pred;
    P_post = P_pred;
end

== matlab function simulator_manual_MPC/Controller/MPC Controller ==
  settings: updateMethod=DISCRETE  sampleTime=dt
  data: x input size=[6, 1]; x_sp input; u output double size=[7 1]; Ad input; Bd input; MPC_settings input
function u = fcn(x, x_sp, Ad, Bd, MPC_settings)
persistent initialized
persistent options

if isempty(initialized)
    %options = optimoptions('quadprog', 'Algorithm', 'active-set');
    %options = optimoptions('quadprog', 'Algorithm', 'fmincon');
    options = optimoptions('fmincon', 'Algorithm','sqp','OptimalityTolerance', 1e-2);
    initialized = true;
end
%x_tilde = [x_sp; zeros(3,1)] - x;
u = MPC(Ad, Bd, x, x_sp, MPC_settings, options);

== matlab function simulator_manual_MPC/Simulator/MATLAB Function ==
  data: q input; qdot input; W input; dLdq_ output; m input; g input; Lh input
function dLdq_ = dLdq_call(q, qdot, W, m, g, Lh)
    temp_struct.W = W;
    temp_struct.m = m;
    temp_struct.g = g;
    temp_struct.L_h = Lh;
    dLdq_ = dLdq(q, qdot, temp_struct);
end

== matlab function simulator_manual_MPC/Controller/R calc ==
  data: q input; R output
function R = fcn(q)
R = Rot_mat(q);

== matlab function simulator_manual_MPC/Controller/Q_abduction ==
  data: f input; Q output; q input; rpli input; rpmi input; R input
function Q = fcn(f, q, rpli, rpmi, R)

Q = Qi(f, q, rpli, rpmi, R);

== matlab function simulator_manual_MPC/Controller/Q_external_rotation_upper ==
  data: f input; Q output; q input; rpli input; rpmi input; R input
function Q = fcn(f, q, rpli, rpmi, R)

Q = Qi(f, q, rpli, rpmi, R);

== matlab function simulator_manual_MPC/Controller/Q_interal_rotation_upper ==
  data: f input; Q output; q input; rpli input; rpmi input; R input
function Q = fcn(f, q, rpli, rpmi, R)

Q = Qi(f, q, rpli, rpmi, R);

== matlab function simulator_manual_MPC/Controller/Q_Extension ==
  data: f input; Q output; q input; rpli input; rpmi input; R input
function Q = fcn(f, q, rpli, rpmi, R)

Q = Qi(f, q, rpli, rpmi, R);

== matlab function simulator_manual_MPC/Controller/Q_Flexion ==
  data: f input; Q output; q input; rpli input; rpmi input; R input
function Q = fcn(f, q, rpli, rpmi, R)

Q = Qi(f, q, rpli, rpmi, R);
